simulink model "systolic_hwcosim"  (R2021a)
settings: Solver=VariableStepAuto  StartTime=0.0  StopTime=100  RelTol=1e-3
undefined symbols (not defined in the file or in its folder): A, N
libraries: hdlBasic x33, xbsIndex_r4 x1, JTAGRuntimeCosim_r4 x1
settings Model: Creator=asc8  LastModifiedBy=asc8

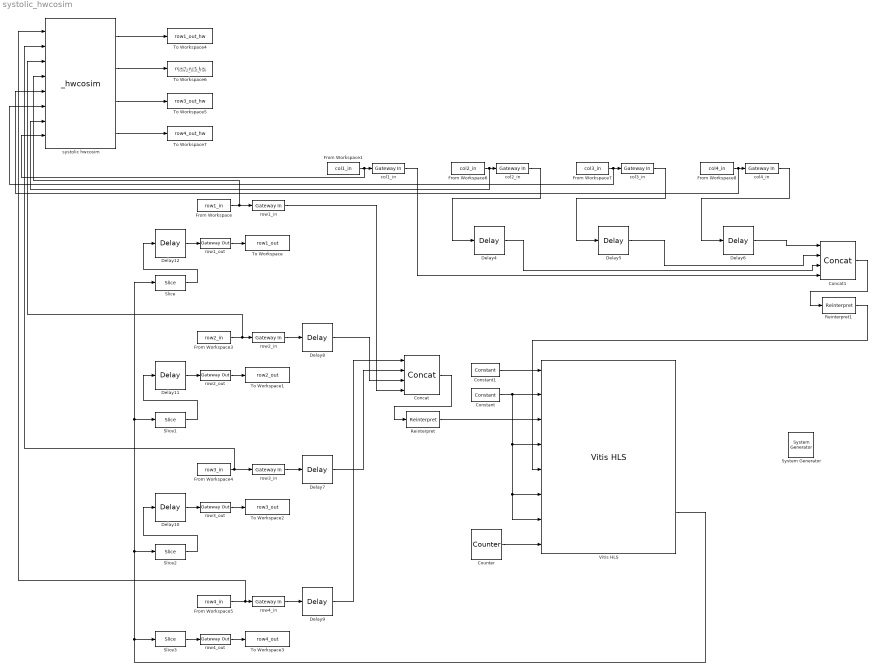
== system systolic_hwcosim ==
  note: row2_out_hw
  " System Generator" : xbsIndex_r4/ System Generator  Tag=genX  xilinxfamily=zynq  part=xc7z020  speed=-1  package=clg484  synthesis_tool=Vivado  clock_wrapper=Clock Enables  directory=./netlist  proj_type=Vivado  Synth_file=Vivado Synthesis Defaults  Impl_file=Vivado Implementation Defaults  testbench=off  simulink_period=1  sysclk_period=2.6387  dcm_input_clock_period=10  incr_netlist=off  trim_vbits=Everywhere in SubSystem  dbl_ovrd=According to Block Masks  core_generation=According to Block Masks  run_coregen=off  deprecated_control=off  eval_field=0  block_type=sysgen
  Concat : hdlBasic/Concat  num_inputs=4  XmcBlockStatus=1  maskContainerNames=group1  block_type=concat  block_config=sysgen:Concat_config
  Concat1 : hdlBasic/Concat  num_inputs=4  XmcBlockStatus=1  maskContainerNames=group1  block_type=concat  block_config=sysgen:Concat_config
  Constant : hdlBasic/Constant  const=1.0  gui_display_data_type=Boolean  arith_type=Boolean  n_bits=16  bin_pt=14  preci_type=Single  exp_width=8  frac_width=24  explicit_period=off  period=1  XmcBlockStatus=1  maskContainerNames=tabcontainer1  block_type=constant  block_config=sysgen:Constant_config
  Constant1 : hdlBasic/Constant  const=0  gui_display_data_type=Boolean  arith_type=Boolean  n_bits=16  bin_pt=14  preci_type=Single  exp_width=8  frac_width=24  explicit_period=off  period=1  XmcBlockStatus=1  maskContainerNames=tabcontainer1  block_type=constant  block_config=sysgen:Constant_config
  Counter : hdlBasic/Counter  cnt_type=Free running  cnt_to=3  operation=Up  start_count=0  cnt_by_val=1  arith_type=Unsigned  n_bits=32  bin_pt=0  load_pin=off  rst=off  en=off  explicit_period=Explicit  period=1  use_behavioral_HDL=off  implementation=Fabric  XmcBlockStatus=1  maskContainerNames=group1  block_type=counter  block_config=sysgen:Counter_config
  Delay10 : hdlBasic/Delay  rst=off  en=off  latency=1  reg_retiming=off  XmcBlockStatus=1  maskContainerNames=group1  block_type=delay  block_config=sysgen:Delay_config
  Delay11 : hdlBasic/Delay  rst=off  en=off  latency=2  reg_retiming=off  XmcBlockStatus=1  maskContainerNames=group1  block_type=delay  block_config=sysgen:Delay_config
  Delay12 : hdlBasic/Delay  rst=off  en=off  latency=3  reg_retiming=off  XmcBlockStatus=1  maskContainerNames=group1  block_type=delay  block_config=sysgen:Delay_config
  Delay4 : hdlBasic/Delay  rst=off  en=off  latency=1  reg_retiming=off  XmcBlockStatus=1  maskContainerNames=group1  block_type=delay  block_config=sysgen:Delay_config
  Delay5 : hdlBasic/Delay  rst=off  en=off  latency=2  reg_retiming=off  XmcBlockStatus=1  maskContainerNames=group1  block_type=delay  block_config=sysgen:Delay_config
  Delay6 : hdlBasic/Delay  rst=off  en=off  latency=3  reg_retiming=off  XmcBlockStatus=1  maskContainerNames=group1  block_type=delay  block_config=sysgen:Delay_config
  Delay7 : hdlBasic/Delay  rst=off  en=off  latency=2  reg_retiming=off  XmcBlockStatus=1  maskContainerNames=group1  block_type=delay  block_config=sysgen:Delay_config
  Delay8 : hdlBasic/Delay  rst=off  en=off  latency=1  reg_retiming=off  XmcBlockStatus=1  maskContainerNames=group1  block_type=delay  block_config=sysgen:Delay_config
  Delay9 : hdlBasic/Delay  rst=off  en=off  latency=3  reg_retiming=off  XmcBlockStatus=1  maskContainerNames=group1  block_type=delay  block_config=sysgen:Delay_config
  From Workspace : FromWorkspace  VariableName=row1_in
  From Workspace1 : FromWorkspace  VariableName=col1_in
  From Workspace3 : FromWorkspace  VariableName=row2_in
  From Workspace4 : FromWorkspace  VariableName=row3_in
  From Workspace5 : FromWorkspace  VariableName=row4_in
  From Workspace6 : FromWorkspace  VariableName=col2_in
  From Workspace7 : FromWorkspace  VariableName=col3_in
  From Workspace8 : FromWorkspace  VariableName=col4_in
  Reinterpret : hdlBasic/Reinterpret  force_arith_type=on  arith_type="Signed  (2's comp)"  force_bin_pt=on  bin_pt=0  XmcBlockStatus=1  maskContainerNames=group1  block_type=reinterpret  block_config=sysgen:Reinterpret_config
  Reinterpret1 : hdlBasic/Reinterpret  force_arith_type=on  arith_type="Signed  (2's comp)"  force_bin_pt=on  bin_pt=0  XmcBlockStatus=1  maskContainerNames=group1  block_type=reinterpret  block_config=sysgen:Reinterpret_config
  Slice : hdlBasic/Slice  nbits=16  boolean_output=off  mode=Upper Bit Location + Width  bit1=-48  base1=MSB of Input  bit0=0  base0=LSB of Input  XmcBlockStatus=1  maskContainerNames=group1  block_type=slice  block_config=sysgen:Slice_config
  Slice1 : hdlBasic/Slice  nbits=16  boolean_output=off  mode=Upper Bit Location + Width  bit1=-32  base1=MSB of Input  bit0=0  base0=LSB of Input  XmcBlockStatus=1  maskContainerNames=group1  block_type=slice  block_config=sysgen:Slice_config
  Slice2 : hdlBasic/Slice  nbits=16  boolean_output=off  mode=Upper Bit Location + Width  bit1=-16  base1=MSB of Input  bit0=0  base0=LSB of Input  XmcBlockStatus=1  maskContainerNames=group1  block_type=slice  block_config=sysgen:Slice_config
  Slice3 : hdlBasic/Slice  nbits=16  boolean_output=off  mode=Upper Bit Location + Width  bit1=0  base1=MSB of Input  bit0=0  base0=LSB of Input  XmcBlockStatus=1  maskContainerNames=group1  block_type=slice  block_config=sysgen:Slice_config
  To Workspace : ToWorkspace  VariableName=row1_out  SaveFormat=Timeseries  SampleTime=-1
  To Workspace1 : ToWorkspace  VariableName=row2_out  SaveFormat=Timeseries  SampleTime=-1
  To Workspace2 : ToWorkspace  VariableName=row3_out  SaveFormat=Timeseries  SampleTime=-1
  To Workspace3 : ToWorkspace  VariableName=row4_out  SaveFormat=Timeseries  SampleTime=-1
  To Workspace4 : ToWorkspace  VariableName=row1_out_hw  SaveFormat=Timeseries  SampleTime=-1
  To Workspace5 : ToWorkspace  VariableName=row3_out_hw  SaveFormat=Timeseries  SampleTime=-1
  To Workspace6 : ToWorkspace  VariableName=row2_out_hw  SaveFormat=Timeseries  SampleTime=-1
  To Workspace7 : ToWorkspace  VariableName=row4_out_hw  SaveFormat=Timeseries  SampleTime=-1
  Vitis HLS : hdlBasic/Vitis HLS  anytable='.\Vitis_HLS\systolicmul\solution1'  fast_sim=off  display_datatype=off  rate_propagation_method=Simulink system period  model_file_path=''  latency=1  block_type=vitis_hls
      settings: infoedit=This block allows including C,C++ and SystemC source files in System Generator for DSP designs.
  col1_in : hdlBasic/Gateway In  gui_display_data_type=Fixed-point  arith_type=Unsigned  n_bits=16  bin_pt=0  preci_type=Single  exp_width=8  frac_width=24  rows=1  columns=1  quantization="Round  (unbiased: +/- Inf)"  overflow=Saturate  period=1  UseAsADC=off  ADCChannel='1'  interface=None  automatic_assignment=on  address_offset=hex2dec('00')  intf_name=''  intf_description=''  default_value=0  timing_constraint=None  locs_specified=off  LOCs={}  io_standard={}  inherit_from_input=off  hdl_port=on  XmcBlockStatus=1  maskContainerNames=group4  block_type=gatewayin  block_config=sysgen:gateway_in_config  block_width_w=590  block_height_w=620  block_width=640  block_height=850
  col2_in : hdlBasic/Gateway In  gui_display_data_type=Fixed-point  arith_type=Unsigned  n_bits=16  bin_pt=0  preci_type=Single  exp_width=8  frac_width=24  rows=1  columns=1  quantization="Round  (unbiased: +/- Inf)"  overflow=Saturate  period=1  UseAsADC=off  ADCChannel='1'  interface=None  automatic_assignment=on  address_offset=hex2dec('00')  intf_name=''  intf_description=''  default_value=0  timing_constraint=None  locs_specified=off  LOCs={}  io_standard={}  inherit_from_input=off  hdl_port=on  XmcBlockStatus=1  maskContainerNames=group4  block_type=gatewayin  block_config=sysgen:gateway_in_config  block_width_w=590  block_height_w=620  block_width=640  block_height=850
  col3_in : hdlBasic/Gateway In  gui_display_data_type=Fixed-point  arith_type=Unsigned  n_bits=16  bin_pt=0  preci_type=Single  exp_width=8  frac_width=24  rows=1  columns=1  quantization="Round  (unbiased: +/- Inf)"  overflow=Saturate  period=1  UseAsADC=off  ADCChannel='1'  interface=None  automatic_assignment=on  address_offset=hex2dec('00')  intf_name=''  intf_description=''  default_value=0  timing_constraint=None  locs_specified=off  LOCs={}  io_standard={}  inherit_from_input=off  hdl_port=on  XmcBlockStatus=1  maskContainerNames=group4  block_type=gatewayin  block_config=sysgen:gateway_in_config  block_width_w=590  block_height_w=620  block_width=640  block_height=850
  col4_in : hdlBasic/Gateway In  gui_display_data_type=Fixed-point  arith_type=Unsigned  n_bits=16  bin_pt=0  preci_type=Single  exp_width=8  frac_width=24  rows=1  columns=1  quantization="Round  (unbiased: +/- Inf)"  overflow=Saturate  period=1  UseAsADC=off  ADCChannel='1'  interface=None  automatic_assignment=on  address_offset=hex2dec('00')  intf_name=''  intf_description=''  default_value=0  timing_constraint=None  locs_specified=off  LOCs={}  io_standard={}  inherit_from_input=off  hdl_port=on  XmcBlockStatus=1  maskContainerNames=group4  block_type=gatewayin  block_config=sysgen:gateway_in_config  block_width_w=590  block_height_w=620  block_width=640  block_height=850
  row1_in : hdlBasic/Gateway In  gui_display_data_type=Fixed-point  arith_type=Unsigned  n_bits=16  bin_pt=0  preci_type=Single  exp_width=8  frac_width=24  rows=1  columns=1  quantization="Round  (unbiased: +/- Inf)"  overflow=Saturate  period=1  UseAsADC=off  ADCChannel='1'  interface=None  automatic_assignment=on  address_offset=hex2dec('00')  intf_name=''  intf_description=''  default_value=0  timing_constraint=None  locs_specified=off  LOCs={}  io_standard={}  inherit_from_input=off  hdl_port=on  XmcBlockStatus=1  maskContainerNames=group4  block_type=gatewayin  block_config=sysgen:gateway_in_config  block_width_w=590  block_height_w=620  block_width=640  block_height=850
  row1_out : hdlBasic/Gateway Out  inherit_from_input=off  hdl_port=on  rows=1  columns=1  UseAsDAC=off  DACChannel='1'  interface=None  automatic_assignment=on  address_offset=hex2dec('00')  intf_name=''  intf_description=''  timing_constraint=None  locs_specified=off  LOCs={}  io_standard={}  XmcBlockStatus=1  maskContainerNames=group4  block_type=gatewayout  block_config=sysgen:gateway_out_config  block_width_w=590  block_height_w=620  block_width=620  block_height=750
  row2_in : hdlBasic/Gateway In  gui_display_data_type=Fixed-point  arith_type=Unsigned  n_bits=16  bin_pt=0  preci_type=Single  exp_width=8  frac_width=24  rows=1  columns=1  quantization="Round  (unbiased: +/- Inf)"  overflow=Saturate  period=1  UseAsADC=off  ADCChannel='1'  interface=None  automatic_assignment=on  address_offset=hex2dec('00')  intf_name=''  intf_description=''  default_value=0  timing_constraint=None  locs_specified=off  LOCs={}  io_standard={}  inherit_from_input=off  hdl_port=on  XmcBlockStatus=1  maskContainerNames=group4  block_type=gatewayin  block_config=sysgen:gateway_in_config  block_width_w=590  block_height_w=620  block_width=640  block_height=850
  row2_out : hdlBasic/Gateway Out  inherit_from_input=off  hdl_port=on  rows=1  columns=1  UseAsDAC=off  DACChannel='1'  interface=None  automatic_assignment=on  address_offset=hex2dec('00')  intf_name=''  intf_description=''  timing_constraint=None  locs_specified=off  LOCs={}  io_standard={}  XmcBlockStatus=1  maskContainerNames=group4  block_type=gatewayout  block_config=sysgen:gateway_out_config  block_width_w=590  block_height_w=620  block_width=620  block_height=750
  row3_in : hdlBasic/Gateway In  gui_display_data_type=Fixed-point  arith_type=Unsigned  n_bits=16  bin_pt=0  preci_type=Single  exp_width=8  frac_width=24  rows=1  columns=1  quantization="Round  (unbiased: +/- Inf)"  overflow=Saturate  period=1  UseAsADC=off  ADCChannel='1'  interface=None  automatic_assignment=on  address_offset=hex2dec('00')  intf_name=''  intf_description=''  default_value=0  timing_constraint=None  locs_specified=off  LOCs={}  io_standard={}  inherit_from_input=off  hdl_port=on  XmcBlockStatus=1  maskContainerNames=group4  block_type=gatewayin  block_config=sysgen:gateway_in_config  block_width_w=590  block_height_w=620  block_width=640  block_height=850
  row3_out : hdlBasic/Gateway Out  inherit_from_input=off  hdl_port=on  rows=1  columns=1  UseAsDAC=off  DACChannel='1'  interface=None  automatic_assignment=on  address_offset=hex2dec('00')  intf_name=''  intf_description=''  timing_constraint=None  locs_specified=off  LOCs={}  io_standard={}  XmcBlockStatus=1  maskContainerNames=group4  block_type=gatewayout  block_config=sysgen:gateway_out_config  block_width_w=590  block_height_w=620  block_width=620  block_height=750
  row4_in : hdlBasic/Gateway In  gui_display_data_type=Fixed-point  arith_type=Unsigned  n_bits=16  bin_pt=0  preci_type=Single  exp_width=8  frac_width=24  rows=1  columns=1  quantization="Round  (unbiased: +/- Inf)"  overflow=Saturate  period=1  UseAsADC=off  ADCChannel='1'  interface=None  automatic_assignment=on  address_offset=hex2dec('00')  intf_name=''  intf_description=''  default_value=0  timing_constraint=None  locs_specified=off  LOCs={}  io_standard={}  inherit_from_input=off  hdl_port=on  XmcBlockStatus=1  maskContainerNames=group4  block_type=gatewayin  block_config=sysgen:gateway_in_config  block_width_w=590  block_height_w=620  block_width=640  block_height=850
  row4_out : hdlBasic/Gateway Out  inherit_from_input=off  hdl_port=on  rows=1  columns=1  UseAsDAC=off  DACChannel='1'  interface=None  automatic_assignment=on  address_offset=hex2dec('00')  intf_name=''  intf_description=''  timing_constraint=None  locs_specified=off  LOCs={}  io_standard={}  XmcBlockStatus=1  maskContainerNames=group4  block_type=gatewayout  block_config=sysgen:gateway_out_config  block_width_w=590  block_height_w=620  block_width=620  block_height=750
  systolic hwcosim : JTAGRuntimeCosim_r4/_hwcosim  clkSrc=Single Stepped  hasCombinationalPath=on  bitfileName=C:\ELEC522\asc8\prj3\netlist\systolic.bit  skipConfig=off  dispPartInfo=off  useZynqReconfigScript=on  cable=Auto Detect  speed=N/A  cablePort=N/A  cableLocation=Local  shareCable=off  xmp=[]  software_settings=[]  design_xtable=|  binDir=[]  engineDll=JTAGCosimEngine.dll  cableWaitTime=10  bscanPos=-1  IRLengths=[]  useWaitBox=1  hasBufgmux=on  Scheme=Cosim  useCmdProc=1  hasProc=0  useImpact=0  printLogFile=0  userChain=2  XmcBlockStatus=0  maskContainerNames=tabcontainer1  block_type=jtagcosim  block_config=Sysgen:hwcosim_block_config
      | {
      |     'clkWrapper' => 'systolic',
      |     'burstMode' => false,
      |     'burstFifoDepth' => '1024',
      |     'shared_memories' => {},
      |     'clocksGcd' => 1,
      |     'device' => {
      |       'family' => 'zynq',
      |       'part' => 'xc7z020',
      |       'package' => 'clg484',
      |       'speed' => '-1',
      |     },
      |     'ports' => {
      |       'row4_in' => {
      |         'direction' => 'in',
      |         'width' => 16,
      |         'name' => 'row4_in',
      |         'period' => 1,
      |         'icon_text' => 'row4_in',
      |         'type' => 'UFix_16_0',
      |         'arithmetic_type' => 'xlUnsigned',
      |         'dat_file' => 'systolic_row4_in.dat',
      |         'bin_pt' => 0,
      |         'addr_offset' => 0,
      |         'bd_port_index' => 0,
      |       },
      |       'row3_in' => {
      |         'direction' => 'in',
      |         'width' => 16,
      |         'name' => 'row3_in',
      |         'period' => 1,
      |         'icon_text' => 'row3_in',
      |         'type' => 'UFix_16_0',
      |         'arithmetic_type' => 'xlUnsigned',
      |         'dat_file' => 'systolic_row3_in.dat',
      |         'bin_pt' => 0,
      |         'addr_offset' => 4,
      |         'bd_port_index' => 1,
      |       },
      |       'row2_in' => {
      |         'direction' => 'in',
      |         'width' => 16,
      |         'name' => 'row2_in',
      |         'period' => 1,
      |         'icon_text' => 'row2_in',
      |         'type' => 'UFix_16_0',
      |         'arithmetic_type' => 'xlUnsigned',
      |         'dat_file' => 'systolic_row2_in.dat',
      |         'bin_pt' => 0,
      |         'addr_offset' => 8,
      |         'bd_port_index' => 2,
      |       },
      |       'row1_in' => {
      |         'direction' => 'in',
      |         'width' => 16,
      |         'name' => 'row1_in',
      |         'period' => 1,
      |         'icon_text' => 'row1_in',
      |         'type' => 'UFix_16_0',
      |         'arithmetic_type' => 'xlUnsigned',
      |         'dat_file' => 'systolic_row1_in.dat',
      |         'bin_pt' => 0,
      |         'addr_offset' => 12,
      |         'bd_port_index' => 3,
      |       },
      |       'col4_in' => {
      |         'direction' => 'in',
      |         'width' => 16,
      |         'name' => 'col4_in',
      |         'period' => 1,
      |         'icon_text' => 'col4_in',
      |         'type' => 'UFix_16_0',
      |         'arithmetic_type' => 'xlUnsigned',
      |         'dat_file' => 'systolic_col4_in.dat',
      |         'bin_pt' => 0,
      |         'addr_offset' => 16,
      |         'bd_port_index' => 4,
      |       },
      |       'col3_in' => {
      |         'direction' => 'in',
      |         'width' => 16,
      |         'name' => 'col3_in',
      |         'period' => 1,
      |         'icon_text' => 'col3_in',
      |         'type' => 'UFix_16_0',
      |         'arithmetic_type' => 'xlUnsigned',
      |         'dat_file' => 'systolic_col3_in.dat',
      |         'bin_pt' => 0,
      |         'addr_offset' => 20,
      |         'bd_port_index' => 5,
      |       },
      |       'col2_in' => {
      |         'direction' => 'in',
      |         'width' => 16,
      |         'name' => 'col2_in',
      |         'period' => 1,
      |         'icon_text' => 'col2_in',
      |         'type' => 'UFix_16_0',
      |         'arithmetic_type' => 'xlUnsigned',
      |         'dat_file' => 'systolic_col2_in.dat',
      |         'bin_pt' => 0,
      |         'addr_offset' => 24,
      |         'bd_port_index' => 6,
      |       },
      |       'col1_in' => {
      |         'direction' => 'in',
      |         'width' => 16,
      |         'name' => 'col1_in',
      |         'period' => 1,
      |         'icon_text' => 'col1_in',
      |         'type' => 'UFix_16_0',
      |         'arithmetic_type' => 'xlUnsigned',
      |         'dat_file' => 'systolic_col1_in.dat',
      |         'bin_pt' => 0,
      |         'addr_offset' => 28,
      |         'bd_port_index' => 7,
      |       },
      |       'row1_out' => {
      |         'direction' => 'out',
      |         'width' => 16,
      |         'name' => 'row1_out',
      |         'period' => 1,
      |         'icon_text' => 'row1_out',
      |         'type' => 'UFix_16_0',
      |         'arithmetic_type' => 'xlUnsigned',
      |         'dat_file' => 'systolic_row1_out.dat',
      |         'bin_pt' => 0,
      |         'addr_offset' => 32,
      |         'bd_port_index' => 0,
      |       },
      |       'row2_out' => {
      |         'direction' => 'out',
      |         'width' => 16,
      |         'name' => 'row2_out',
      |         'period' => 1,
      |         'icon_text' => 'row2_out',
      |         'type' => 'UFix_16_0',
      |         'arithmetic_type' => 'xlUnsigned',
      |         'dat_file' => 'systolic_row2_out.dat',
      |         'bin_pt' => 0,
      |         'addr_offset' => 36,
      |         'bd_port_index' => 1,
      |       },
      |       'row3_out' => {
      |         'direction' => 'out',
      |         'width' => 16,
      |         'name' => 'row3_out',
      |         'period' => 1,
      |         'icon_text' => 'row3_out',
      |         'type' => 'UFix_16_0',
      |         'arithmetic_type' => 'xlUnsigned',
      |         'dat_file' => 'systolic_row3_out.dat',
      |         'bin_pt' => 0,
      |         'addr_offset' => 40,
      |         'bd_port_index' => 2,
      |       },
      |       'row4_out' => {
      |         'direction' => 'out',
      |         'width' => 16,
      |         'name' => 'row4_out',
      |         'period' => 1,
      |         'icon_text' => 'row4_out',
      |         'type' => 'UFix_16_0',
      |         'arithmetic_type' => 'xlUnsigned',
      |         'dat_file' => 'systolic_row4_out.dat',
      |         'bin_pt' => 0,
      |         'addr_offset' => 44,
      |         'bd_port_index' => 3,
      |       },
      |     },
      |   }
  wires:
  From Workspace/1 -> systolic hwcosim/4, row1_in/1
  row1_out/1 -> To Workspace/1
  From Workspace1/1 -> systolic hwcosim/8, col1_in/1
  From Workspace3/1 -> row2_in/1, systolic hwcosim/3
  row2_out/1 -> To Workspace1/1
  From Workspace4/1 -> systolic hwcosim/2, row3_in/1
  row3_out/1 -> To Workspace2/1
  From Workspace5/1 -> systolic hwcosim/1, row4_in/1
  row4_out/1 -> To Workspace3/1
  From Workspace6/1 -> systolic hwcosim/7, col2_in/1
  From Workspace7/1 -> systolic hwcosim/6, col3_in/1
  From Workspace8/1 -> systolic hwcosim/5, col4_in/1
  col2_in/1 -> Delay4/1
  col3_in/1 -> Delay5/1
  col4_in/1 -> Delay6/1
  row2_in/1 -> Delay8/1
  row3_in/1 -> Delay7/1
  row4_in/1 -> Delay9/1
  Delay10/1 -> row3_out/1
  Delay11/1 -> row2_out/1
  Delay12/1 -> row1_out/1
  Counter/1 -> Vitis HLS/8
  Constant/1 -> Vitis HLS/2, Vitis HLS/4, Vitis HLS/7, Vitis HLS/6
  Constant1/1 -> Vitis HLS/1
  Slice/1 -> Delay12/1
  Slice1/1 -> Delay11/1
  Slice2/1 -> Delay10/1
  Slice3/1 -> row4_out/1
  Vitis HLS/6 -> Slice3/1, Slice/1, Slice1/1, Slice2/1
  Reinterpret/1 -> Vitis HLS/3
  Reinterpret1/1 -> Vitis HLS/5
  Concat/1 -> Reinterpret/1
  Concat1/1 -> Reinterpret1/1
  row1_in/1 -> Concat/4
  Delay8/1 -> Concat/3
  Delay7/1 -> Concat/2
  Delay9/1 -> Concat/1
  col1_in/1 -> Concat1/4
  Delay4/1 -> Concat1/3
  Delay5/1 -> Concat1/2
  Delay6/1 -> Concat1/1
  systolic hwcosim/1 -> To Workspace4/1
  systolic hwcosim/2 -> To Workspace6/1
  systolic hwcosim/3 -> To Workspace5/1
  systolic hwcosim/4 -> To Workspace7/1
